simulink model "finalProject"  (R2018b)
settings: Solver=VariableStepAuto  StartTime=0.0  StopTime=6000  RelTol=1e-3
undefined symbols (not defined in the file): quatMult
libraries: simulink x1
settings Model: Creator=Eric  LastModifiedBy=Eric
settings DebuggingCC: UnderSpecifiedDimensionMsg=warning

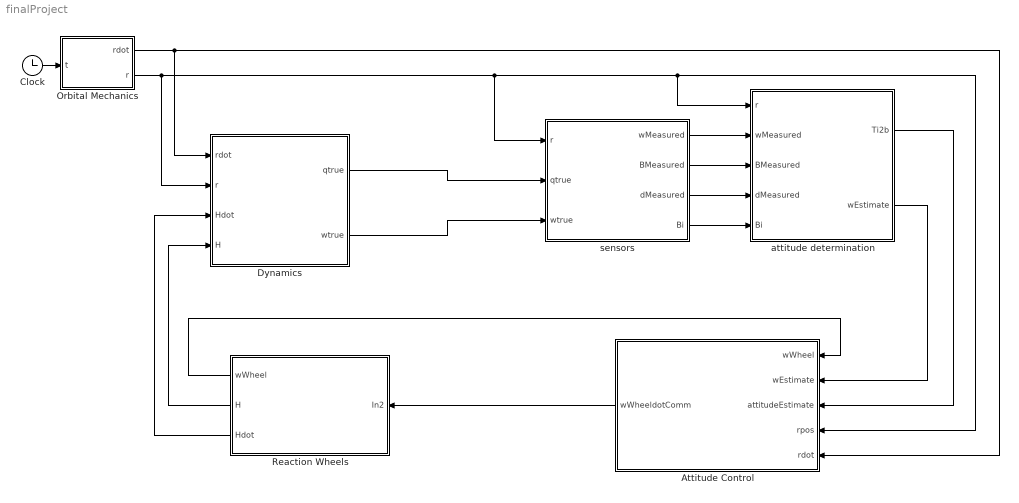
== system finalProject ==
  Attitude Control : MATLAB Function  TreatAsAtomicUnit=on
  Clock : Clock
  Dynamics : Subsystem
  Orbital Mechanics : MATLAB Function  TreatAsAtomicUnit=on
  Reaction Wheels : Subsystem
  attitude determination : MATLAB Function  TreatAsAtomicUnit=on
  sensors : Subsystem
  wires:
  Clock/1 -> Orbital Mechanics/1(t)
  Orbital Mechanics/1(rdot) -> Dynamics/1(rdot), Attitude Control/5(rdot)
  attitude determination/2(wEstimate) -> Attitude Control/2(wEstimate)
  attitude determination/1(Ti2b) -> Attitude Control/3(attitudeEstimate)
  Orbital Mechanics/2(r) -> Dynamics/2(r), sensors/1(r), attitude determination/1(r), Attitude Control/4(rpos)
  sensors/2(BMeasured) -> attitude determination/3(BMeasured)
  Dynamics/1(qtrue) -> sensors/2(qtrue)
  Dynamics/2(wtrue) -> sensors/3(wtrue)
  sensors/1(wMeasured) -> attitude determination/2(wMeasured)
  sensors/3(dMeasured) -> attitude determination/4(dMeasured)
  sensors/4(Bi) -> attitude determination/5(Bi)
  Attitude Control/1(wWheeldotComm) -> Reaction Wheels/1(In2)
  Reaction Wheels/2(H) -> Dynamics/4("H ")
  Reaction Wheels/1(wWheel) -> Attitude Control/1(wWheel)
  Reaction Wheels/3("Hdot ") -> Dynamics/3(Hdot)

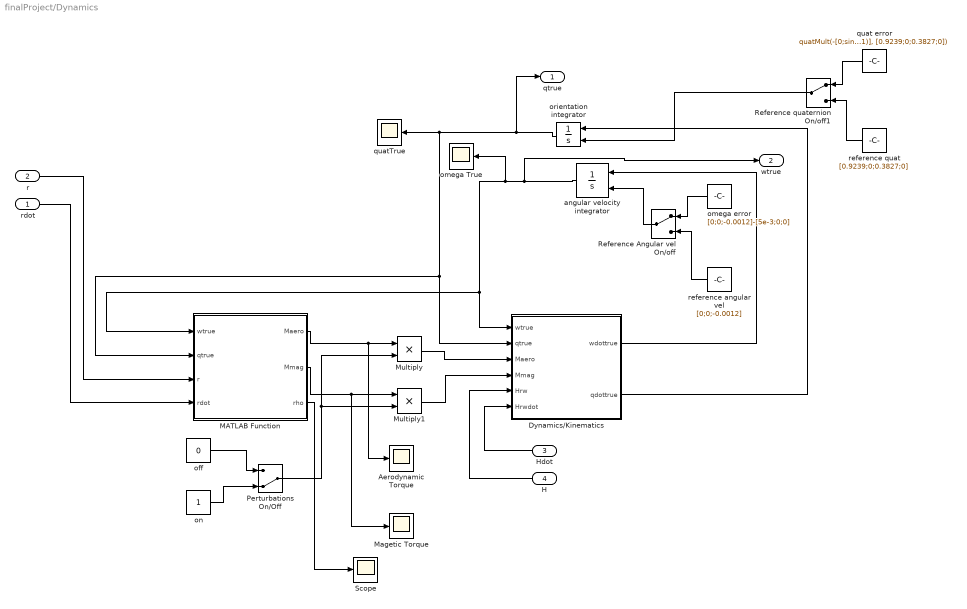
== system finalProject/Dynamics ==
  rdot : Inport
  r : Inport  Port=2
  Hdot : Inport  Port=3
  "H " : Inport  Port=4
  Aerodynamic Torque : Scope
  Dynamics/Kinematics : MATLAB Function  TreatAsAtomicUnit=on
  MATLAB Function : MATLAB Function  TreatAsAtomicUnit=on
  Magetic Torque : Scope
  Multiply : Product
  Multiply1 : Product
  Perturbations On/Off : ManualSwitch  CurrentSetting=0
  Reference Angular vel On/off : ManualSwitch
  Reference quaternion On/off1 : ManualSwitch
  Scope : Scope
  angular velocity integrator : Integrator  InitialConditionSource=external  InitialCondition=[0;0;-0.0012]+[5e-3;0;0]
  off : Constant  Value=0
  omega True : Scope
  omega error : Constant  Value=[0;0;-0.0012]-[5e-3;0;0]
  on : Constant
  orientation integrator : Integrator  InitialConditionSource=external  InitialCondition=quatMult([0;sind(1);0;cosd(1)], [0.9239;0;0.3827;0])
  quat error : Constant  Value=quatMult(-[0;sind(1);0;cosd(1)], [0.9239;0;0.3827;0])
  "quatTrue " : Scope
  reference angular vel : Constant  Value=[0;0;-0.0012]
  reference quat : Constant  Value=[0.9239;0;0.3827;0]
  qtrue : Outport
  wtrue : Outport  Port=2
  wires:
  Dynamics/Kinematics/1(wdottrue) -> angular velocity integrator/1
  Dynamics/Kinematics/2(qdottrue) -> orientation integrator/1
  Hdot/1 -> Dynamics/Kinematics/6(Hrwdot)
  "H "/1 -> Dynamics/Kinematics/5(Hrw)
  orientation integrator/1 -> Dynamics/Kinematics/2(qtrue), MATLAB Function/2(qtrue), "quatTrue "/1, qtrue/1
  angular velocity integrator/1 -> wtrue/1, Dynamics/Kinematics/1(wtrue), MATLAB Function/1(wtrue), omega True/1
  r/1 -> MATLAB Function/3(r)
  rdot/1 -> MATLAB Function/4(rdot)
  MATLAB Function/1(Maero) -> Aerodynamic Torque/1, Multiply/1
  Multiply/1 -> Dynamics/Kinematics/3(Maero)
  MATLAB Function/2(Mmag) -> Magetic Torque/1, Multiply1/1
  Multiply1/1 -> Dynamics/Kinematics/4(Mmag)
  on/1 -> Perturbations On/Off/2
  off/1 -> Perturbations On/Off/1
  Perturbations On/Off/1 -> Multiply1/2, Multiply/2
  reference angular vel/1 -> Reference Angular vel On/off/2
  omega error/1 -> Reference Angular vel On/off/1
  Reference Angular vel On/off/1 -> angular velocity integrator/2
  reference quat/1 -> Reference quaternion On/off1/2
  quat error/1 -> Reference quaternion On/off1/1
  Reference quaternion On/off1/1 -> orientation integrator/2
  MATLAB Function/3(rho) -> Scope/1

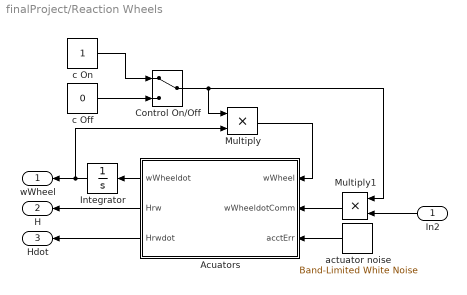
== system finalProject/Reaction Wheels ==
  In2 : Inport
  Acuators : MATLAB Function  TreatAsAtomicUnit=on
  Control On/Off : ManualSwitch
  Integrator : Integrator  InitialCondition=[6.92;6.92;6.92]
  Multiply : Product
  Multiply1 : Product
  actuator noise : simulink/Sources/Band-Limited White Noise  Cov=(pi/5000)^2*[1;1;1]  Ts=0.1  seed=[23341]
  c Off : Constant  Value=0
  c On : Constant
  wWheel : Outport
  H : Outport  Port=2
  "Hdot " : Outport  Port=3
  wires:
  Acuators/1(wWheeldot) -> Integrator/1
  Integrator/1 -> Multiply/2, wWheel/1
  Acuators/2(Hrw) -> H/1
  Acuators/3(Hrwdot) -> "Hdot "/1
  c Off/1 -> Control On/Off/2
  Control On/Off/1 -> Multiply1/1, Multiply/1
  c On/1 -> Control On/Off/1
  Multiply1/1 -> Acuators/2(wWheeldotComm)
  In2/1 -> Multiply1/2
  actuator noise/1 -> Acuators/3(acctErr)
  Multiply/1 -> Acuators/1(wWheel)

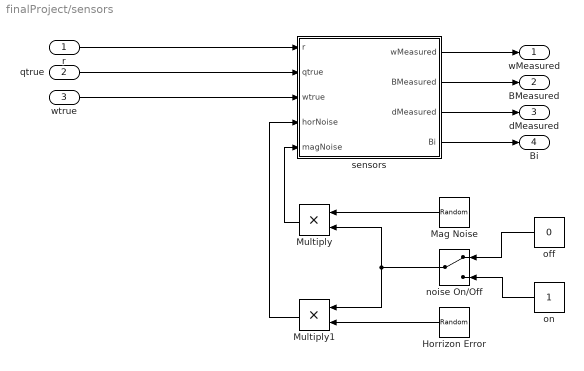
== system finalProject/sensors ==
  r : Inport
  qtrue : Inport  Port=2
  wtrue : Inport  Port=3
  Horrizon Error : RandomNumber  Mean=[0;0;0]  Variance=(pi/180/3)^2*[1;1;1]  Seed=56844
  Mag Noise : RandomNumber  Mean=[0;0;0]  Variance=(.1e-5)^2*[1;1;1]  Seed=1234
  Multiply : Product
  Multiply1 : Product
  noise On/Off : ManualSwitch
  off : Constant  Value=0
  on : Constant
  "sensors " : MATLAB Function  TreatAsAtomicUnit=on
  wMeasured : Outport
  BMeasured : Outport  Port=2
  dMeasured : Outport  Port=3
  Bi : Outport  Port=4
  wires:
  "sensors "/3(dMeasured) -> dMeasured/1
  r/1 -> "sensors "/1(r)
  wtrue/1 -> "sensors "/3(wtrue)
  qtrue/1 -> "sensors "/2(qtrue)
  "sensors "/2(BMeasured) -> BMeasured/1
  Multiply/1 -> "sensors "/5(magNoise)
  "sensors "/4(Bi) -> Bi/1
  "sensors "/1(wMeasured) -> wMeasured/1
  Multiply1/1 -> "sensors "/4(horNoise)
  Horrizon Error/1 -> Multiply1/2
  Mag Noise/1 -> Multiply/1
  off/1 -> noise On/Off/1
  on/1 -> noise On/Off/2
  noise On/Off/1 -> Multiply/2, Multiply1/1

== matlab function finalProject/sensors/sensors  ==
  data: r input; qtrue input; wMeasured output; wtrue input; BMeasured output; dMeasured output; horNoise input; Bi output; magNoise input
function [wMeasured, BMeasured, dMeasured, Bi] = sensors(r, qtrue, wtrue, horNoise, magNoise)

%
%GYRO
%

%https://www.northropgrumman.com/Capabilities/LN200FOG/Documents/ln200s.pdf
%gyro bias = 1degree/hour = 9.696E-6 rad/s
gyroBias = 9.696E-6*[1; 1; 1];
%walk = .07 deg/sqrt(hr)
gyroWalk = (.0012*pi/180)^2*[1;1;1];
wMeasured = wtrue + gyroBias + gyroWalk;
qv = qtrue(2:4);
qs = qtrue(1);

skewv = [0, -qv(3), qv(2); 
         qv(3), 0, -qv(1); 
         -qv(2), qv(1), 0];
    
Ti2b = eye(3) - 2*qs*skewv + 2*skewv*skewv;

%
%MAGNETOMETER
%
Bo = 3.12E-5;
Re = 6371; %km

%DCM inertial to NEZ;
nz = -r/norm(r);
ny = (cross(nz, [0; 0; 1]))/norm(cross(nz, [0; 0; 1]));
nx = cross(ny, nz);
Ti2ned = [ nx'; ny'; nz'];
lambda = asin(r(3)/norm(r));

%magnetic field calculation
Bn = Bo*((Re/norm(r))^3)*[cos(lambda); 0; -2*sin(lambda)];
Bi = Ti2ned'*Bn; 
BMeasured = Ti2b*Bi + magNoise;
BMeasured =  BMeasured/norm(BMeasured);

%
%Horizon
%
horErrT = theta2T(horNoise);
dMeasured = horErrT*Ti2b*(-r/norm(r));
end

function T = theta2T(theta)

nt = norm(theta);
T = eye(3);

if nt > 1e-10
    S = skew(theta/nt);
    T = T - sin(nt)*S + (1-cos(nt))*S^2;
end
end

function S = skew(v)
S = [0 -v(3) v(2);
     v(3) 0 -v(1);
    -v(2) v(1) 0];
end

== matlab function finalProject/Dynamics/MATLAB Function ==
  data: wtrue input; qtrue input; r input; Maero output; rdot input; Mmag output; rho output
function [Maero, Mmag, rho] = Perturbations(wtrue, qtrue, r, rdot)
%
%AERODYNAMIC TORQUE
%
rSwrtCG = [1.2; 0; 0]; %[m]
A = 10; %m^2
Cd = 5;
wE = [0; 0; 7.2921158553E-5];
v = rdot*1000 + cross(wtrue,rSwrtCG) - cross(wE, r*1000); %m/s
Nhat = r/norm(r);
vhat = v/norm(v);

%Exponential Atmospheric Model
H = 268;
rho0 = 3.019E-15;
rho = rho0*exp(-(norm(r)-1000)/H);

%torque calculation
fAero = -.5*Cd*rho*(norm(v)^2)*dot(Nhat,vhat)*vhat*A;
Maero = cross(rSwrtCG, fAero);

%
%MAGNETIC TORQUE
%
mSC = [100;0;0]; %magnetic feild of the spacecraft
Bo = 3.12E-5;
Re = 6371; %km

qv = qtrue(2:4);
qs = qtrue(1);

skewv = [0, -qv(3), qv(2); 
         qv(3), 0, -qv(1); 
         -qv(2), qv(1), 0];
    
Ti2b = eye(3) - 2*qs*skewv + 2*skewv*skewv;

%DCM inertial to NEZ;
nz = -r/norm(r);
ny = (cross(nz, [0; 0; 1]))/norm(cross(nz, [0; 0; 1]));
nx = cross(ny, nz);
Ti2ned = [ nx'; ny'; nz'];
lambda = asin(r(3)/norm(r));

%magnetic field calculation
Bn = Bo*((Re/norm(r))^3)*[cos(lambda); 0; -2*sin(lambda)];
Bi = Ti2ned'*Bn; 
Bb = Ti2b*Bi;

Mmag = cross(mSC,Bb);
end

== matlab function finalProject/Dynamics/Dynamics//Kinematics ==
  data: wdottrue output; wtrue input; qtrue input; Maero input; Mmag input; Hrw input; qdottrue output; Hrwdot input
function [ wdottrue, qdottrue] = dynamics(wtrue, qtrue, Maero, Mmag, Hrw, Hrwdot)
Jcg = [1000, 0, 0; 0, 500, 0; 0, 0, 600];


%
%ATTITUDE PROPAGATION
%
wdottrue = inv(Jcg)*(-cross(wtrue,Jcg*wtrue+Hrw) - Hrwdot + Maero + Mmag);

qwtrue = [0; wtrue];
qdottrue = .5*quatMult(qtrue, qwtrue);

end

== matlab function finalProject/Reaction Wheels/Acuators ==
  data: wWheel input; wWheeldot output; Hrw output; Hrwdot output; wWheeldotComm input; acctErr input
function [wWheeldot, Hrw, Hrwdot] = acuators( wWheel, wWheeldotComm, acctErr)
%acctErr = (.5)*rand(3,1);

wWheeldot = wWheeldotComm + acctErr;

%reaction wheel specs
%http://bluecanyontech.com/rw4/
mw = 3; %kg
r = .17; %m
h = .07; %m
A = (1/12)*mw*(3*r^2 + h^2); 
C = .5*mw*r^2;

Hrwdot = C*wWheeldot;
Hrw = C*wWheel;

== matlab function finalProject/Attitude Control ==
  data: wWheel input; wEstimate input; wWheeldotComm output; attitudeEstimate input; rpos input; rdot input
function wWheeldotComm  = attControl( wWheel, wEstimate, attitudeEstimate, rpos, rdot)
%reaction wheel specs
%http://bluecanyontech.com/rw4/
mw = 3; %kg
r = .17; %m
C = .5*mw*r^2;

JcgS = [1000, 0, 0; 0, 500, 0; 0, 0, 600];

%
%DESIRED ATTITUDE AND RATE
%
mu = 398600.4415; %km
rho = 6600; %km
w = sqrt(mu/rho^3);
wdesired = [0; 0; -w];

xbar = -rpos/norm(rpos);
zbar = cross(xbar, rdot);
zbar = zbar/norm(zbar);
ybar = cross(zbar, xbar);

desiredAtt = [xbar'; ybar'; zbar'];


%
%REACTION WHEEL COMMAND
%

attdot = attitudeEstimate*desiredAtt';
err = -.5*[attdot(3,2) - attdot(2,3); 
           attdot(1,3) - attdot(3,1); 
           attdot(2,1) - attdot(1,2)];

dw =  wEstimate - wdesired;
skewWDesired = [0,         -wdesired(3), wdesired(2);
                wdesired(3), 0,         -wdesired(1);
                -wdesired(2), wdesired(1), 0];
errdot = -skewWDesired*err + dw;
Kd = .8;
Kp = .8;

wWheeldotComm = ((Kp*JcgS)/C)*err + ((Kd*JcgS)/C)*errdot - cross(wEstimate, wWheel);

== matlab function finalProject/Orbital Mechanics ==
  data: rdot output; t input; r output
function [rdot, r] = fcn(t)
mu = 398600.4415;
rho = 6600; %km

w = sqrt(mu/rho^3);
r = (rho/sqrt(2))*[-cos(w*t); sqrt(2)*sin(w*t); cos(w*t)];
rdot = ((w*rho)/(sqrt(2)))*[sin(w*t); sqrt(2)*cos(w*t); -sin(w*t)];

== matlab function finalProject/attitude determination ==
  data: Ti2b output; r input; wEstimate output; wMeasured input; BMeasured input; dMeasured input; Bi input
function [Ti2b, wEstimate] = fcn(r, wMeasured, BMeasured, dMeasured, Bi)


%
%GYRO 
%

wEstimate = wMeasured;

%
%TRIAD
%


d1b = dMeasured;
d2b = BMeasured;

xb = d1b;
zb = cross(d1b, d2b)/norm(cross(d1b, d2b));
yb = cross(zb, xb);

d1i = -r/norm(r);
d2i = Bi/norm(Bi);

xi = d1i;
zi = cross(d1i, d2i)/norm(cross(d1i, d2i));
yi = cross(zi, xi);

Ti2b = [xb, yb, zb]*[xi, yi, zi]';
